simulink model "Utkarsh_2005574_W1_P2"  (R2020b)
settings: Solver=VariableStepAuto  StartTime=0.0  StopTime=100  RelTol=1e-3
PostLoadFcn:
  | m1=2000;
  | m2=80;
  | k1=50;
  | k2=50;
  | b=50;
InitFcn:
  | m1=2000;
  | m2=80;
  | k1=50;
  | k2=50;
  | b=50;
settings Model: Creator=home  LastModifiedBy=home

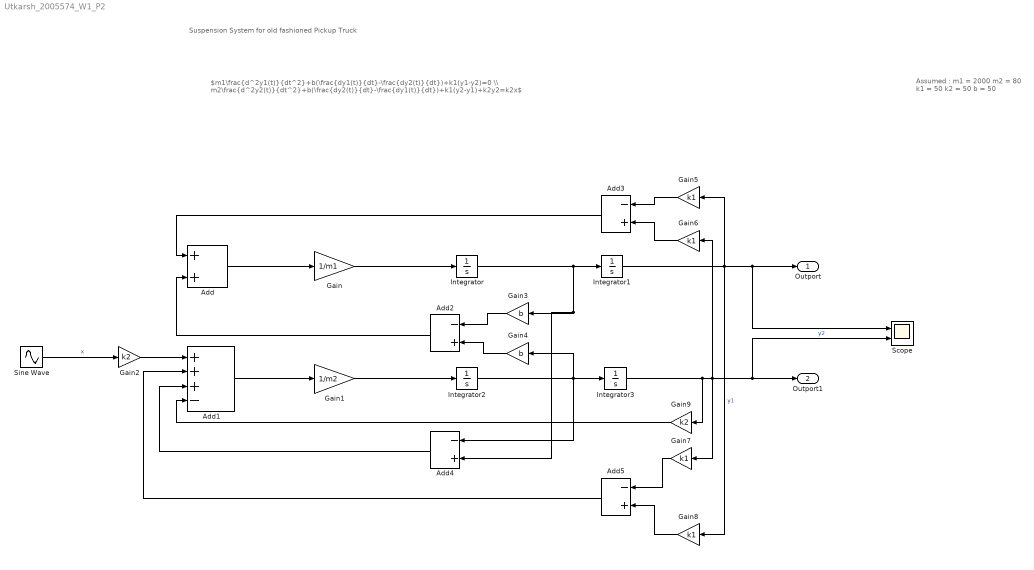
== system Utkarsh_2005574_W1_P2 ==
  note: Assumed :
      | m1 = 2000
      | m2 = 80
      | k1 = 50
      | k2 = 50
      | b = 50
  note: Suspension System for old fashioned Pickup Truck
  note: $m1\frac{d^2y1(t)}{dt^2}+b(\frac{dy1(t)}{dt}-\frac{dy2(t)}{dt})+k1(y1-y2)=0 \\ m2\frac{d^2y2(t)}{dt^2}+b(\frac{dy2(t)}{dt}-\frac{dy1(t)}{dt})+k1(y2-y1)+k2y2=k2x$
  Add : Sum
  Add1 : Sum  Inputs=+++-
  Add{2..5} (4 alike) : Sum  Inputs=-+
  Gain : Gain  Gain=1/m1
  Gain1 : Gain  Gain=1/m2
  Gain2 : Gain  Gain=k2
  Gain3 : Gain  Gain=b
  Gain4 : Gain  Gain=b
  Gain{5..8} (4 alike) : Gain  Gain=k1
  Gain9 : Gain  Gain=k2
  Integrator{,1..3} (4 alike) : Integrator
  Scope : Scope  NumInputPorts=2
  Sine Wave : Sin  Frequency=10  SampleTime=0
  Outport : Outport
  Outport1 : Outport  Port=2
  wires:
  Add/1 -> Gain/1
  Gain/1 -> Integrator/1
  Integrator/1 -> Add4/2, Gain3/1, Integrator1/1
  Integrator1/1 -> Gain8/1, Gain5/1, Scope/1, Outport/1  "y1"
  Add1/1 -> Gain1/1
  Gain1/1 -> Integrator2/1
  Integrator2/1 -> Gain4/1, Integrator3/1, Add4/1
  Integrator3/1 -> Gain9/1, Gain7/1, Scope/2, Outport1/1, Gain6/1  "y2"
  Gain2/1 -> Add1/1
  Sine Wave/1 -> Gain2/1  "x"
  Gain3/1 -> Add2/1
  Gain4/1 -> Add2/2
  Gain5/1 -> Add3/1
  Gain6/1 -> Add3/2
  Add2/1 -> Add/2
  Add3/1 -> Add/1
  Gain8/1 -> Add5/2
  Gain7/1 -> Add5/1
  Gain9/1 -> Add1/4
  Add4/1 -> Add1/3
  Add5/1 -> Add1/2
